simulink model "Simulacion_mayor_a_0"  (R2021b)
settings: Solver=VariableStepAuto  StartTime=0.0  StopTime=10.0  RelTol=1e-3
settings Model: Creator=fer63  LastModifiedBy=fer63

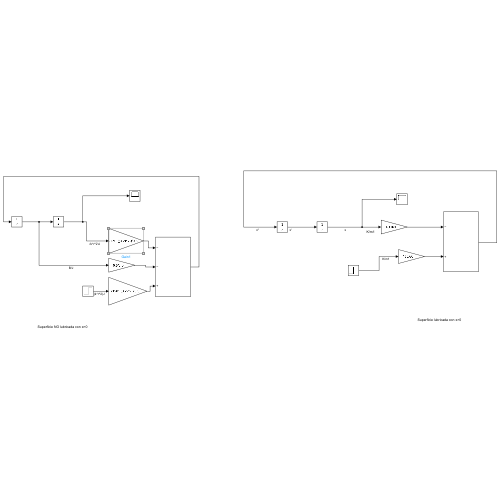
[thumbnail: Simulink's stored preview of the top-level diagram]
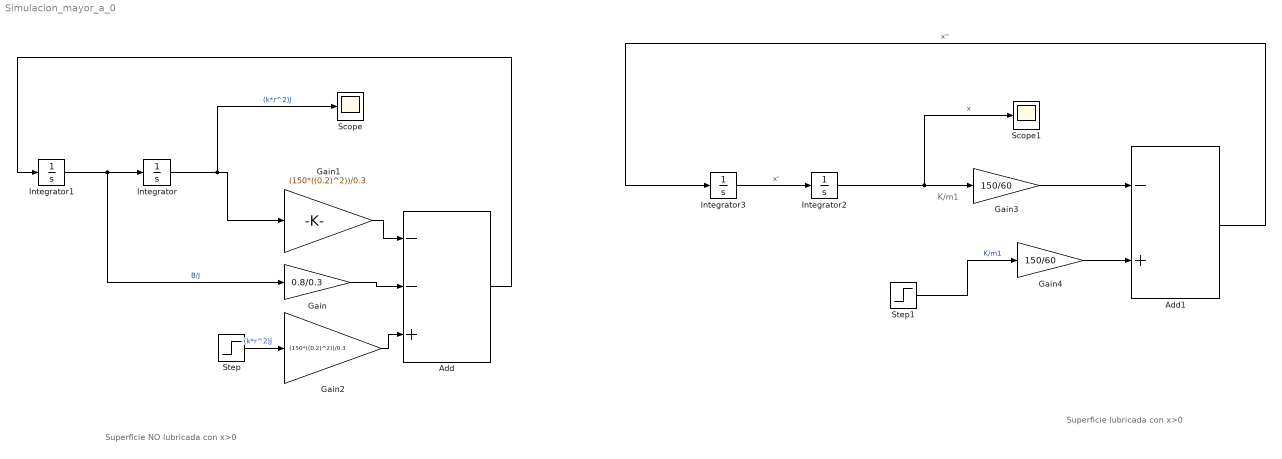
== system Simulacion_mayor_a_0 ==
  note: K/m1
  note: Superficie NO lubricada con x>0
  note: Superficie lubricada con x>0
  Add : Sum  Inputs=--+
  Add1 : Sum  Inputs=-+
  Gain : Gain  Gain=0.8/0.3
  Gain1 : Gain  Gain=(150*((0.2)^2))/0.3
  Gain2 : Gain  Gain=(150*((0.2)^2))/0.3
  Gain3 : Gain  Gain=150/60
  Gain4 : Gain  Gain=150/60
  Integrator{,1..3} (4 alike) : Integrator
  Scope : Scope
  Scope1 : Scope
  Step : Step  Time=0  SampleTime=0
  Step1 : Step  Time=0  SampleTime=0
  wires:
  Gain1/1 -> Add/1
  Gain/1 -> Add/2
  Gain2/1 -> Add/3
  Step/1 -> Gain2/1  "(k*r^2)J"
  Integrator1/1 -> Gain/1, Integrator/1  "B/J"
  Integrator/1 -> Scope/1, Gain1/1  "(k*r^2)J"
  Add/1 -> Integrator1/1
  Gain3/1 -> Add1/1
  Integrator3/1 -> Integrator2/1  "x'"
  Add1/1 -> Integrator3/1  "x''"
  Integrator2/1 -> Scope1/1, Gain3/1  "x"
  Gain4/1 -> Add1/2
  Step1/1 -> Gain4/1  "K/m1"
